simulink model "Copy_of_UAV"  (R2018b)
settings: Solver=FixedStepAuto  StartTime=0  StopTime=300  MaxStep=0.01  RelTol=1e-4  EnableMultiTasking=on
values from neighbouring files (symbols this model uses):
  actuatorCentres = 0.0    [data.sldd]
  datcom1 : value not decoded    [data.sldd]
  deflectionLimits = -10.0    [data.sldd]
  loggingSampleTime = 1.0    [data.sldd]
  sensorSampleTime = 0.02    [data.sldd]
  vehicle = 1.5    [data.sldd]
undefined symbols (not defined in the file or in its folder): aeroCoeff, DiscIntNeverNeededParam, Discrete, HDBK, MIL, Time
libraries: simulink x24, arduinolib x8, ctrlSharedLib x8, aerolibasang x5, aerolibactuator x4, aerolibadyn x3, aerolibconvert2 x2, aerolibatmos2 x2, aerolibnav x2, shared6dof x1, aerolibwind2 x1, simulink_extras x1
(part 2 of 3)

== system Copy_of_UAV/Flight Dynamics/Coeff Model/Aerodynamic Coefficients/Body Rate Damping ==
  V : Inport  Unit=m/s
  Bus Element In : Inport  Port=2  PortName=pqr  Element=p_wind
  Bus Element In1 : Inport  Port=2  PortName=pqr  Element=q_wind
  Bus Element In2 : Inport  Port=2  PortName=pqr  Element=r_wind
  Product : Product  SaturateOnIntegerOverflow=on  InputSameDT=on  OutDataTypeStr=Inherit: Same as first input
  Product1 : Product  SaturateOnIntegerOverflow=on  InputSameDT=on  OutDataTypeStr=Inherit: Same as first input
  Product2 : Product  SaturateOnIntegerOverflow=on  InputSameDT=on  OutDataTypeStr=Inherit: Same as first input
  Product3 : Product  Inputs=*/  SaturateOnIntegerOverflow=on  InputSameDT=on  OutDataTypeStr=Inherit: Same as first input
  Reference Length : Gain  Gain=vehicle.chord  SaturateOnIntegerOverflow=on  OutDataTypeStr=Inherit: Same as input  ParamDataTypeStr=Inherit: Same as input
  Reference Span : Gain  Gain=vehicle.wingspan/2  SaturateOnIntegerOverflow=on  OutDataTypeStr=Inherit: Same as input  ParamDataTypeStr=Inherit: Same as input
  "Reference Span " : Gain  Gain=vehicle.wingspan/2  SaturateOnIntegerOverflow=on  OutDataTypeStr=Inherit: Same as input  ParamDataTypeStr=Inherit: Same as input
  Sum1 : Sum  Inputs=+++  SaturateOnIntegerOverflow=on  InputSameDT=on  OutDataTypeStr=Inherit: Same as first input
  p : Subsystem
  q : Subsystem
  r : Subsystem
  Coeff : Outport  InitialOutput=0
  wires:
  Bus Element In/1 -> Product/2
  Bus Element In1/1 -> Product1/2
  Bus Element In2/1 -> Product2/2
  p/1(delCoeff) -> Product/1
  q/1(delCoeff) -> Product1/1
  Sum1/1 -> Product3/1
  V/1 -> Product3/2
  Product3/1 -> Coeff/1
  Product1/1 -> Reference Length/1
  Product2/1 -> "Reference Span "/1
  Product/1 -> Reference Span/1
  r/1(delCoeff) -> Product2/1
  Reference Length/1 -> Sum1/2
  Reference Span/1 -> Sum1/1
  "Reference Span "/1 -> Sum1/3

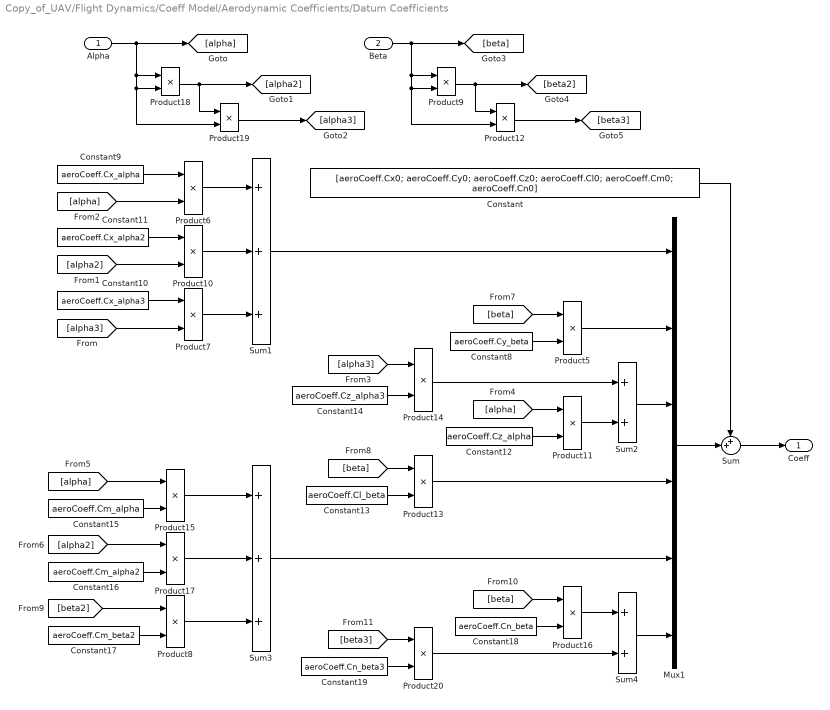
== system Copy_of_UAV/Flight Dynamics/Coeff Model/Aerodynamic Coefficients/Datum Coefficients ==
  Alpha : Inport
  Beta : Inport  Port=2
  Constant : Constant  Value=[aeroCoeff.Cx0; aeroCoeff.Cy0; aeroCoeff.Cz0; aeroCoeff.Cl0; aeroCoeff.Cm0; aeroCoeff.Cn0]
  Constant10 : Constant  Value=aeroCoeff.Cx_alpha3
  Constant11 : Constant  Value=aeroCoeff.Cx_alpha2
  Constant12 : Constant  Value=aeroCoeff.Cz_alpha
  Constant13 : Constant  Value=aeroCoeff.Cl_beta
  Constant14 : Constant  Value=aeroCoeff.Cz_alpha3
  Constant15 : Constant  Value=aeroCoeff.Cm_alpha
  Constant16 : Constant  Value=aeroCoeff.Cm_alpha2
  Constant17 : Constant  Value=aeroCoeff.Cm_beta2
  Constant18 : Constant  Value=aeroCoeff.Cn_beta
  Constant19 : Constant  Value=aeroCoeff.Cn_beta3
  Constant8 : Constant  Value=aeroCoeff.Cy_beta
  Constant9 : Constant  Value=aeroCoeff.Cx_alpha
  Mux1 : Mux  Inputs=6
  Product{5..20} (16 alike) : Product  SaturateOnIntegerOverflow=on  InputSameDT=on  OutDataTypeStr=Inherit: Same as first input
  Sum : Sum  Inputs=++|
  Sum1 : Sum  Inputs=+++  SaturateOnIntegerOverflow=on
  Sum2 : Sum  Inputs=2  SaturateOnIntegerOverflow=on
  Sum3 : Sum  Inputs=+++  SaturateOnIntegerOverflow=on
  Sum4 : Sum  Inputs=2  SaturateOnIntegerOverflow=on
  Coeff : Outport  InitialOutput=0
  wires:
  Sum/1 -> Coeff/1
  Constant/1 -> Sum/1
  Mux1/1 -> Sum/2
  Sum3/1 -> Mux1/5
  Product16/1 -> Sum4/1
  Product20/1 -> Sum4/2
  [beta3] -> Product20/1
  [beta] -> Product16/1
  Constant19/1 -> Product20/2
  Constant18/1 -> Product16/2
  Sum4/1 -> Mux1/6
  [beta2] -> Product8/1
  [beta] -> Product13/1
  [beta] -> Product5/1
  Beta/1 -> Product9/1, Product12/2, Product9/2, [beta]
  Product9/1 -> Product12/1, [beta2]
  Product12/1 -> [beta3]
  Product8/1 -> Sum3/3
  Constant17/1 -> Product8/2
  [alpha] -> Product15/1
  [alpha] -> Product11/1
  [alpha3] -> Product14/1
  [alpha] -> Product6/2
  [alpha2] -> Product10/2
  Constant10/1 -> Product7/1
  [alpha3] -> Product7/2
  Product19/1 -> [alpha3]
  Product18/1 -> [alpha2], Product19/1
  Alpha/1 -> [alpha], Product18/2, Product19/2, Product18/1
  Constant16/1 -> Product17/2
  Product17/1 -> Sum3/2
  [alpha2] -> Product17/1
  Constant15/1 -> Product15/2
  Product15/1 -> Sum3/1
  Constant14/1 -> Product14/2
  Product13/1 -> Mux1/4
  Constant13/1 -> Product13/2
  Sum2/1 -> Mux1/3
  Product14/1 -> Sum2/1
  Product11/1 -> Sum2/2
  Constant12/1 -> Product11/2
  Product10/1 -> Sum1/2
  Product6/1 -> Sum1/1
  Product7/1 -> Sum1/3
  Constant11/1 -> Product10/1
  Constant9/1 -> Product6/1
  Sum1/1 -> Mux1/1
  Product5/1 -> Mux1/2
  Constant8/1 -> Product5/2

== system Copy_of_UAV/Flight Dynamics/DATCOM Model/Aero Coeffs/Aileron ==
  Bus : Inport
  Bus Selector2 : BusSelector  OutputSignals=idxa,fa,idxda,fda,idxm,fm,idxh,fh
  Bus Selector3 : BusSelector  OutputSignals=idxda,fda,idxm,fm,idxh,fh
  Constant1 : Constant  Value=0
  DCL_Roll : Interpolation_n-D  NumberOfTableDimensions=3  Table="permute(datcom1{2}.clroll,[1  2  3])"  RemoveProtectionIndex=on
      settings: InputPortMap=u0,u1,u2,u3,u4,u5
  DCN_Asym : Interpolation_n-D  NumberOfTableDimensions=4  Table=permute(datcom1{2}.cn_asy,[1 2 3 4 ])  RemoveProtectionIndex=on
      settings: InputPortMap=u0,u1,u2,u3,u4,u5,u6,u7
  Mux1 : Mux  Inputs=6
  delCoeff : Outport
  wires:
  Mux1/1 -> delCoeff/1
  Bus Selector3/5 -> DCL_Roll/5  "<idxh>"
  Constant1/1 -> Mux1/1, Mux1/2, Mux1/3, Mux1/5
  Bus Selector3/4 -> DCL_Roll/4  "<fm>"
  Bus Selector3/3 -> DCL_Roll/3  "<idxm>"
  Bus Selector3/6 -> DCL_Roll/6  "<fh>"
  Bus Selector3/1 -> DCL_Roll/1  "<idxda>"
  Bus Selector3/2 -> DCL_Roll/2  "<fda>"
  Bus Selector2/2 -> DCN_Asym/2  "<fa>"
  Bus Selector2/1 -> DCN_Asym/1  "<idxa>"
  Bus/1 -> Bus Selector2/1, Bus Selector3/1
  Bus Selector2/3 -> DCN_Asym/3  "<idxda>"
  Bus Selector2/4 -> DCN_Asym/4  "<fda>"
  Bus Selector2/5 -> DCN_Asym/5  "<idxm>"
  Bus Selector2/6 -> DCN_Asym/6  "<fm>"
  Bus Selector2/7 -> DCN_Asym/7  "<idxh>"
  Bus Selector2/8 -> DCN_Asym/8  "<fh>"
  DCN_Asym/1 -> Mux1/6
  DCL_Roll/1 -> Mux1/4

== system Copy_of_UAV/Flight Dynamics/DATCOM Model/Aero Coeffs/Elevator ==
  Bus : Inport
  Bus Selector2 : BusSelector  OutputSignals=idxa,fa,idxm,fm,idxh,fh,idxde,fde
  Bus Selector3 : BusSelector  OutputSignals=idxde,fde,idxm,fm,idxh,fh
  Bus Selector5 : BusSelector  OutputSignals=idxde,fde,idxm,fm,idxh,fh
  Constant1 : Constant  Value=0
  DCDI : Interpolation_n-D  NumberOfTableDimensions=4  Table=permute(datcom1{3}.dcdi_sym,[1 3 4 2 ])  RemoveProtectionIndex=on
      settings: InputPortMap=u0,u1,u2,u3,u4,u5,u6,u7
  DCL : Interpolation_n-D  NumberOfTableDimensions=3  Table="permute(datcom1{3}.dcl_sym,[1  2  3])"  RemoveProtectionIndex=on
      settings: InputPortMap=u0,u1,u2,u3,u4,u5
  DCm : Interpolation_n-D  NumberOfTableDimensions=3  Table="permute(datcom1{3}.dcm_sym,[1  2  3])"  RemoveProtectionIndex=on
      settings: InputPortMap=u0,u1,u2,u3,u4,u5
  Mux1 : Mux  Inputs=6
  delCoeff : Outport
  wires:
  Mux1/1 -> delCoeff/1
  Bus/1 -> Bus Selector2/1, Bus Selector3/1, Bus Selector5/1
  DCDI/1 -> Mux1/1
  DCL/1 -> Mux1/3
  DCm/1 -> Mux1/5
  Constant1/1 -> Mux1/2, Mux1/4, Mux1/6
  Bus Selector2/1 -> DCDI/1  "<idxa>"
  Bus Selector2/2 -> DCDI/2  "<fa>"
  Bus Selector3/1 -> DCL/1  "<idxde>"
  Bus Selector3/2 -> DCL/2  "<fde>"
  Bus Selector5/1 -> DCm/1  "<idxde>"
  Bus Selector5/2 -> DCm/2  "<fde>"
  Bus Selector2/3 -> DCDI/3  "<idxm>"
  Bus Selector2/4 -> DCDI/4  "<fm>"
  Bus Selector2/5 -> DCDI/5  "<idxh>"
  Bus Selector2/6 -> DCDI/6  "<fh>"
  Bus Selector2/7 -> DCDI/7  "<idxde>"
  Bus Selector2/8 -> DCDI/8  "<fde>"
  Bus Selector3/3 -> DCL/3  "<idxm>"
  Bus Selector3/4 -> DCL/4  "<fm>"
  Bus Selector3/5 -> DCL/5  "<idxh>"
  Bus Selector3/6 -> DCL/6  "<fh>"
  Bus Selector5/3 -> DCm/3  "<idxm>"
  Bus Selector5/4 -> DCm/4  "<fm>"
  Bus Selector5/5 -> DCm/5  "<idxh>"
  Bus Selector5/6 -> DCm/6  "<fh>"

== system Copy_of_UAV/Flight Dynamics/DATCOM Model/Aero Coeffs/Rudder ==
  Bus : Inport
  Constant1 : Constant  Value=0
  Mux1 : Mux  Inputs=6
  Terminator : Terminator
  delCoeff : Outport
  wires:
  Mux1/1 -> delCoeff/1
  Constant1/1 -> Mux1/6, Mux1/5, Mux1/4, Mux1/3, Mux1/2, Mux1/1
  Bus/1 -> Terminator/1

== system Copy_of_UAV/Primary Arduino/Flight Control/Model Flight Control/Guidance/Guidance.ALT_Hold.ALT ==
  Sensors : Inport  OutDataTypeStr=Bus: Sensors
  Demands : Inport  Port=2  OutDataTypeStr=Bus: Demands
  Control Override : Inport  Port=3  OutDataTypeStr=Bus: ControlOverrides
  Action Port : ActionPort
      settings: CopyFcn=Stateflow.SLINSF.SimulinkMan.removeBlockPreDeleteFcn  PreDeleteFcn=Stateflow.SLINSF.SimulinkMan.unsafePredeleteFcn
  Altitude Hold : Subsystem
  Bus Selector : BusSelector  OutputSignals=Altitude,phi_theta_psi
  Bus Selector1 : BusSelector  OutputSignals=Altitude
  Bus Selector2 : BusSelector  OutputSignals=Aileron
  Mux : Mux  Inputs=2
  Rate Limiter : RateLimiter  SampleTimeMode=inherited
  Selector2 : Selector  IndexMode=Zero-based  InputPortWidth=3  IndexOptions=Index vector (dialog)  Indices=[1]  OutputSizes=1
  Commands : Outport
  wires:
  Mux/1 -> Commands/1
  Altitude Hold/1(Elevator) -> Mux/2
  Selector2/1 -> Altitude Hold/3(theta)
  Sensors/1 -> Bus Selector/1
  Demands/1 -> Bus Selector1/1
  Bus Selector/1 -> Altitude Hold/1(ALT)  "<Altitude>"
  Bus Selector/2 -> Selector2/1  "<phi_theta_psi>"
  Bus Selector1/1 -> Rate Limiter/1  "<Altitude>"
  Rate Limiter/1 -> Altitude Hold/2(Demanded ALT)
  Bus Selector2/1 -> Mux/1  "<Aileron>"
  Control Override/1 -> Bus Selector2/1

== system Copy_of_UAV/Primary Arduino/Flight Control/Model Flight Control/Guidance/Guidance.HDG_ALT_Hold.HDG_ALT ==
  Sensors : Inport  OutDataTypeStr=Bus: Sensors
  Demands : Inport  Port=2  OutDataTypeStr=Bus: Demands
  Action Port : ActionPort
      settings: CopyFcn=Stateflow.SLINSF.SimulinkMan.removeBlockPreDeleteFcn  PreDeleteFcn=Stateflow.SLINSF.SimulinkMan.unsafePredeleteFcn
  Altitude Hold : Subsystem
      settings: UndoDeleteFcn=Stateflow.SLINSF.SimulinkMan.restorePreDeleteFcn  PreDeleteFcn=Stateflow.SLINSF.SimulinkMan.removePreDeleteFcn
  Bus Selector : BusSelector  OutputSignals=Heading,phi_theta_psi,Altitude
  Bus Selector1 : BusSelector  OutputSignals=Heading,Altitude
  Heading Hold : Subsystem
  Mux : Mux  Inputs=2
  Rate Limiter : RateLimiter  SampleTimeMode=inherited
  Rate Limiter1 : RateLimiter  SampleTimeMode=inherited
  Selector : Selector  IndexMode=Zero-based  InputPortWidth=3  IndexOptions=Index vector (dialog)  Indices=[0]  OutputSizes=1
  Selector2 : Selector  IndexMode=Zero-based  InputPortWidth=3  IndexOptions=Index vector (dialog)  Indices=[1]  OutputSizes=1
  Commands : Outport
  wires:
  Heading Hold/1(Aileron) -> Mux/1  "Aileron"
  Mux/1 -> Commands/1
  Altitude Hold/1(Elevator) -> Mux/2  "Elevator"
  Selector2/1 -> Altitude Hold/3(theta)
  Sensors/1 -> Bus Selector/1
  Selector/1 -> Heading Hold/3(Current Roll Angle)
  Demands/1 -> Bus Selector1/1
  Bus Selector/3 -> Altitude Hold/1(ALT)  "<Altitude>"
  Bus Selector1/1 -> Rate Limiter/1  "<Heading>"
  Bus Selector/1 -> Heading Hold/1(Current Heading)  "<Heading>"
  Bus Selector/2 -> Selector2/1, Selector/1  "<phi_theta_psi>"
  Bus Selector1/2 -> Rate Limiter1/1  "<Altitude>"
  Rate Limiter/1 -> Heading Hold/2(Demanded Heading)
  Rate Limiter1/1 -> Altitude Hold/2(ALT Demand)

== system Copy_of_UAV/Primary Arduino/Flight Control/Model Flight Control/Guidance/Guidance.HDG_Hold.HDG ==
  Sensors : Inport  OutDataTypeStr=Bus: Sensors
  Demands : Inport  Port=2  OutDataTypeStr=Bus: Demands
  Control Override : Inport  Port=3  OutDataTypeStr=Bus: ControlOverrides
  Action Port : ActionPort
      settings: CopyFcn=Stateflow.SLINSF.SimulinkMan.removeBlockPreDeleteFcn  PreDeleteFcn=Stateflow.SLINSF.SimulinkMan.unsafePredeleteFcn
  Bus Selector : BusSelector  OutputSignals=Heading,phi_theta_psi
  Bus Selector1 : BusSelector  OutputSignals=Heading
  Bus Selector2 : BusSelector  OutputSignals=Elevator
  Heading Hold : Subsystem
  Mux : Mux  Inputs=2
  Rate Limiter : RateLimiter  SampleTimeMode=inherited
  Selector : Selector  IndexMode=Zero-based  InputPortWidth=3  IndexOptions=Index vector (dialog)  Indices=[0]  OutputSizes=1
  Command : Outport
  wires:
  Heading Hold/1(Aileron Command) -> Mux/1  "Aileron"
  Sensors/1 -> Bus Selector/1
  Selector/1 -> Heading Hold/3(Current Roll Angle)
  Demands/1 -> Bus Selector1/1
  Bus Selector1/1 -> Rate Limiter/1  "<Heading>"
  Bus Selector/1 -> Heading Hold/1(Current Heading)  "<Heading>"
  Bus Selector/2 -> Selector/1  "<phi_theta_psi>"
  Rate Limiter/1 -> Heading Hold/2(Demanded Heading)
  Mux/1 -> Command/1
  Control Override/1 -> Bus Selector2/1
  Bus Selector2/1 -> Mux/2  "<Elevator>"

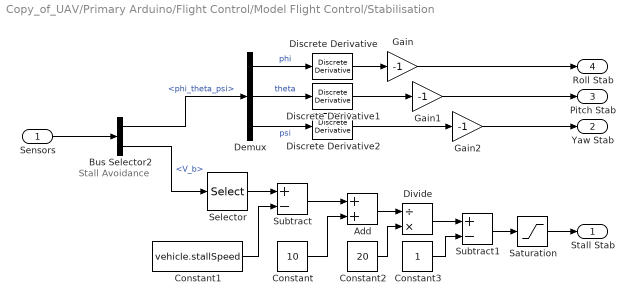
== system Copy_of_UAV/Primary Arduino/Flight Control/Model Flight Control/Stabilisation ==
  note: Stall Avoidance
  Sensors : Inport
  Add : Sum
  Bus Selector2 : BusSelector  OutputSignals=phi_theta_psi,V_b
  Constant : Constant  Value=10  OutDataTypeStr=single
  Constant1 : Constant  Value=vehicle.stallSpeed  OutDataTypeStr=single
  Constant2 : Constant  Value=20  OutDataTypeStr=single
  Constant3 : Constant  OutDataTypeStr=single
  Demux : Demux  Outputs=3
  Discrete Derivative : simulink/Discrete/Discrete Derivative  gainval=1.0  ICPrevScaledInput=0.0  OutMin=[]  OutMax=[]  OutDataType=fixdt(1, 16)  OutScaling=2^-10  DoSatur=off
  Discrete Derivative1 : simulink/Discrete/Discrete Derivative  gainval=1.0  ICPrevScaledInput=0.0  OutMin=[]  OutMax=[]  OutDataType=fixdt(1, 16)  OutScaling=2^-10  DoSatur=off
  Discrete Derivative2 : simulink/Discrete/Discrete Derivative  gainval=1.0  ICPrevScaledInput=0.0  OutMin=[]  OutMax=[]  OutDataType=fixdt(1, 16)  OutScaling=2^-10  DoSatur=off
  Divide : Product  Inputs=/*
  Gain : Gain  Gain=-1
  Gain1 : Gain  Gain=-1
  Gain2 : Gain  Gain=-1
  Saturation : Saturate  UpperLimit=1  LowerLimit=0
  Selector : Selector  IndexMode=Zero-based  InputPortWidth=3  IndexOptions=Index vector (dialog)  Indices=[0]  OutputSizes=1
  Subtract : Sum  Inputs=+-
  Subtract1 : Sum  Inputs=+-
  Stall Stab : Outport
  Yaw Stab : Outport  Port=2
  Pitch Stab : Outport  Port=3
  Roll Stab : Outport  Port=4
  wires:
  Gain2/1 -> Yaw Stab/1
  Bus Selector2/2 -> Selector/1  "<V_b>"
  Discrete Derivative2/1 -> Gain2/1
  Selector/1 -> Subtract/1
  Sensors/1 -> Bus Selector2/1
  Demux/2 -> Discrete Derivative1/1  "theta"
  Demux/1 -> Discrete Derivative/1  "phi"
  Demux/3 -> Discrete Derivative2/1  "psi"
  Discrete Derivative1/1 -> Gain1/1
  Discrete Derivative/1 -> Gain/1
  Bus Selector2/1 -> Demux/1  "<phi_theta_psi>"
  Gain/1 -> Roll Stab/1
  Gain1/1 -> Pitch Stab/1
  Constant1/1 -> Subtract/2
  Saturation/1 -> Stall Stab/1
  Subtract/1 -> Add/1
  Constant/1 -> Add/2
  Add/1 -> Divide/1
  Constant2/1 -> Divide/2
  Divide/1 -> Subtract1/1
  Constant3/1 -> Subtract1/2
  Subtract1/1 -> Saturation/1

== system Copy_of_UAV/Primary Arduino/Flight Control/Real Flight Control/Guidance/Guidance.ALT_Hold.ALT ==
  Sensors : Inport  OutDataTypeStr=Bus: Sensors
  Demands : Inport  Port=2  OutDataTypeStr=Bus: Demands
  Action Port : ActionPort
      settings: CopyFcn=Stateflow.SLINSF.SimulinkMan.removeBlockPreDeleteFcn  PreDeleteFcn=Stateflow.SLINSF.SimulinkMan.unsafePredeleteFcn
  Altitude Hold : Subsystem
  Bus Selector : BusSelector  OutputSignals=Altitude,phi_theta_psi
  Bus Selector1 : BusSelector  OutputSignals=Altitude
  Constant : Constant  Value=0
  Mux : Mux  Inputs=2
  Rate Limiter : RateLimiter  SampleTimeMode=inherited
  Selector2 : Selector  IndexMode=Zero-based  InputPortWidth=3  IndexOptions=Index vector (dialog)  Indices=[1]  OutputSizes=1
  Commands : Outport
  wires:
  Mux/1 -> Commands/1
  Altitude Hold/1(Elevator) -> Mux/2
  Selector2/1 -> Altitude Hold/3(theta)
  Sensors/1 -> Bus Selector/1
  Demands/1 -> Bus Selector1/1
  Bus Selector/1 -> Altitude Hold/1(ALT)  "<Altitude>"
  Bus Selector/2 -> Selector2/1  "<phi_theta_psi>"
  Bus Selector1/1 -> Rate Limiter/1  "<Altitude>"
  Rate Limiter/1 -> Altitude Hold/2(Demanded ALT)
  Constant/1 -> Mux/1

== system Copy_of_UAV/Primary Arduino/Flight Control/Real Flight Control/Guidance/Guidance.HDG_ALT_Hold.HDG_ALT ==
  Sensors : Inport  OutDataTypeStr=Bus: Sensors
  Demands : Inport  Port=2  OutDataTypeStr=Bus: Demands
  Action Port : ActionPort
      settings: CopyFcn=Stateflow.SLINSF.SimulinkMan.removeBlockPreDeleteFcn  PreDeleteFcn=Stateflow.SLINSF.SimulinkMan.unsafePredeleteFcn
  Altitude Hold : Subsystem
      settings: UndoDeleteFcn=Stateflow.SLINSF.SimulinkMan.restorePreDeleteFcn  PreDeleteFcn=Stateflow.SLINSF.SimulinkMan.removePreDeleteFcn
  Bus Selector : BusSelector  OutputSignals=Heading,phi_theta_psi,Altitude
  Bus Selector1 : BusSelector  OutputSignals=Heading,Altitude
  Heading Hold : Subsystem
  Mux : Mux  Inputs=2
  Rate Limiter : RateLimiter  SampleTimeMode=inherited
  Rate Limiter1 : RateLimiter  SampleTimeMode=inherited
  Selector : Selector  IndexMode=Zero-based  InputPortWidth=3  IndexOptions=Index vector (dialog)  Indices=[0]  OutputSizes=1
  Selector2 : Selector  IndexMode=Zero-based  InputPortWidth=3  IndexOptions=Index vector (dialog)  Indices=[1]  OutputSizes=1
  Commands : Outport
  wires:
  Heading Hold/1(Aileron) -> Mux/1  "Aileron"
  Mux/1 -> Commands/1
  Altitude Hold/1(Elevator) -> Mux/2  "Elevator"
  Selector2/1 -> Altitude Hold/3(theta)
  Sensors/1 -> Bus Selector/1
  Selector/1 -> Heading Hold/3(Current Roll Angle)
  Demands/1 -> Bus Selector1/1
  Bus Selector/3 -> Altitude Hold/1(ALT)  "<Altitude>"
  Bus Selector1/1 -> Rate Limiter/1  "<Heading>"
  Bus Selector/1 -> Heading Hold/1(Current Heading)  "<Heading>"
  Bus Selector/2 -> Selector2/1, Selector/1  "<phi_theta_psi>"
  Bus Selector1/2 -> Rate Limiter1/1  "<Altitude>"
  Rate Limiter/1 -> Heading Hold/2(Demanded Heading)
  Rate Limiter1/1 -> Altitude Hold/2(ALT Demand)

== system Copy_of_UAV/Primary Arduino/Flight Control/Real Flight Control/Guidance/Guidance.HDG_Hold.HDG ==
  Sensors : Inport  OutDataTypeStr=Bus: Sensors
  Demands : Inport  Port=2  OutDataTypeStr=Bus: Demands
  Action Port : ActionPort
      settings: CopyFcn=Stateflow.SLINSF.SimulinkMan.removeBlockPreDeleteFcn  PreDeleteFcn=Stateflow.SLINSF.SimulinkMan.unsafePredeleteFcn
  Bus Selector : BusSelector  OutputSignals=Heading,phi_theta_psi
  Bus Selector1 : BusSelector  OutputSignals=Heading
  Constant : Constant  Value=0
  Heading Hold : Subsystem
  Mux : Mux  Inputs=2
  Rate Limiter : RateLimiter  SampleTimeMode=inherited
  Selector : Selector  IndexMode=Zero-based  InputPortWidth=3  IndexOptions=Index vector (dialog)  Indices=[0]  OutputSizes=1
  Command : Outport
  wires:
  Heading Hold/1(Aileron Command) -> Mux/1  "Aileron"
  Sensors/1 -> Bus Selector/1
  Selector/1 -> Heading Hold/3(Current Roll Angle)
  Demands/1 -> Bus Selector1/1
  Bus Selector1/1 -> Rate Limiter/1  "<Heading>"
  Bus Selector/1 -> Heading Hold/1(Current Heading)  "<Heading>"
  Bus Selector/2 -> Selector/1  "<phi_theta_psi>"
  Rate Limiter/1 -> Heading Hold/2(Demanded Heading)
  Mux/1 -> Command/1
  Constant/1 -> Mux/2

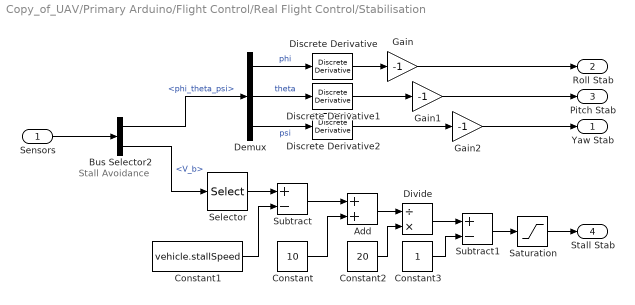
== system Copy_of_UAV/Primary Arduino/Flight Control/Real Flight Control/Stabilisation ==
  note: Stall Avoidance
  Sensors : Inport
  Add : Sum
  Bus Selector2 : BusSelector  OutputSignals=phi_theta_psi,V_b
  Constant : Constant  Value=10  OutDataTypeStr=single
  Constant1 : Constant  Value=vehicle.stallSpeed  OutDataTypeStr=single
  Constant2 : Constant  Value=20  OutDataTypeStr=single
  Constant3 : Constant  OutDataTypeStr=single
  Demux : Demux  Outputs=3
  Discrete Derivative : simulink/Discrete/Discrete Derivative  gainval=1.0  ICPrevScaledInput=0.0  OutMin=[]  OutMax=[]  OutDataType=fixdt(1, 16)  OutScaling=2^-10  DoSatur=off
  Discrete Derivative1 : simulink/Discrete/Discrete Derivative  gainval=1.0  ICPrevScaledInput=0.0  OutMin=[]  OutMax=[]  OutDataType=fixdt(1, 16)  OutScaling=2^-10  DoSatur=off
  Discrete Derivative2 : simulink/Discrete/Discrete Derivative  gainval=1.0  ICPrevScaledInput=0.0  OutMin=[]  OutMax=[]  OutDataType=fixdt(1, 16)  OutScaling=2^-10  DoSatur=off
  Divide : Product  Inputs=/*
  Gain : Gain  Gain=-1
  Gain1 : Gain  Gain=-1
  Gain2 : Gain  Gain=-1
  Saturation : Saturate  UpperLimit=1  LowerLimit=0
  Selector : Selector  IndexMode=Zero-based  InputPortWidth=3  IndexOptions=Index vector (dialog)  Indices=[0]  OutputSizes=1
  Subtract : Sum  Inputs=+-
  Subtract1 : Sum  Inputs=+-
  Yaw Stab : Outport
  Roll Stab : Outport  Port=2
  Pitch Stab : Outport  Port=3
  Stall Stab : Outport  Port=4
  wires:
  Gain2/1 -> Yaw Stab/1
  Bus Selector2/2 -> Selector/1  "<V_b>"
  Discrete Derivative2/1 -> Gain2/1
  Selector/1 -> Subtract/1
  Sensors/1 -> Bus Selector2/1
  Demux/2 -> Discrete Derivative1/1  "theta"
  Demux/1 -> Discrete Derivative/1  "phi"
  Demux/3 -> Discrete Derivative2/1  "psi"
  Discrete Derivative1/1 -> Gain1/1
  Discrete Derivative/1 -> Gain/1
  Bus Selector2/1 -> Demux/1  "<phi_theta_psi>"
  Gain/1 -> Roll Stab/1
  Gain1/1 -> Pitch Stab/1
  Constant1/1 -> Subtract/2
  Saturation/1 -> Stall Stab/1
  Subtract/1 -> Add/1
  Constant/1 -> Add/2
  Add/1 -> Divide/1
  Constant2/1 -> Divide/2
  Divide/1 -> Subtract1/1
  Constant3/1 -> Subtract1/2
  Subtract1/1 -> Saturation/1

== system Copy_of_UAV/Primary Arduino/Sensors/Sensor Hardware/Model Sensors ==
  States : Inport
  Add : Sum
  "BMP280 PAT Sensor " : Subsystem
  Bus Selector : BusSelector  OutputSignals=X_e,phi_theta_psi,pqr,A_be,omega_dot
  Constant2 : Constant  Value=9.81  OutDataTypeStr=single
  Constant3 : Constant  Value=vehicle.CG  OutDataTypeStr=single
  Constant4 : Constant  OutDataTypeStr=single
  Divide1 : Product  Inputs=*/
  L3GD20 3 Axis Gyro Sensor : Subsystem
  LSM303 Accel + Compass Sensor : Subsystem
  Pressure_Pa : Outport
  Temp_C : Outport  Port=2
  RotVel : Outport  Port=3
  LinAccel : Outport  Port=4
  Heading : Outport  Port=5
  Altitude : Outport  Port=6
  wires:
  Constant3/1 -> LSM303 Accel + Compass Sensor/4(CoG)
  Constant4/1 -> Add/2
  Bus Selector/1 -> "BMP280 PAT Sensor "/1(X_e)  "<X_e>"
  Constant2/1 -> Divide1/2
  Bus Selector/4 -> LSM303 Accel + Compass Sensor/1(A_b), Divide1/1  "<A_be>"
  Bus Selector/3 -> LSM303 Accel + Compass Sensor/2(omega), L3GD20 3 Axis Gyro Sensor/1(omega)  "<pqr>"
  L3GD20 3 Axis Gyro Sensor/1(RotVel) -> RotVel/1  "RotVel"
  Add/1 -> L3GD20 3 Axis Gyro Sensor/2(G's)
  Divide1/1 -> Add/1
  "BMP280 PAT Sensor "/3(Altitude_m) -> Altitude/1  "Altitude"
  Bus Selector/2 -> LSM303 Accel + Compass Sensor/5(phi_theta_psi)  "<phi_theta_psi>"
  Bus Selector/5 -> LSM303 Accel + Compass Sensor/3(omega_dot)  "<omega_dot>"
  LSM303 Accel + Compass Sensor/1(LinAccel) -> LinAccel/1  "LinAccel"
  "BMP280 PAT Sensor "/1(Pressure_Pa) -> Pressure_Pa/1  "Pressure_Pa"
  States/1 -> Bus Selector/1
  "BMP280 PAT Sensor "/2(Temp_C) -> Temp_C/1  "Temp_C"
  LSM303 Accel + Compass Sensor/2(hdg_deg) -> Heading/1  "Heading"

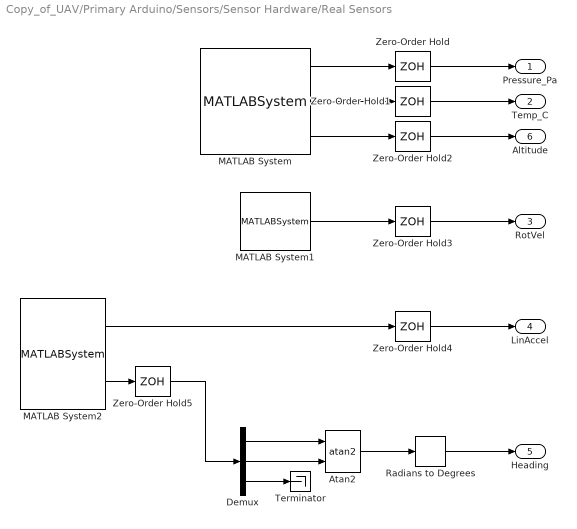
== system Copy_of_UAV/Primary Arduino/Sensors/Sensor Hardware/Real Sensors ==
  Atan2 : Trigonometry  Operator=atan2
  Demux : Demux  Outputs=3
  MATLAB System : MATLABSystem  System=BMP085  Reference_Pressure=101325  SimulateUsing=Code generation
      mask Type: BMP085
      mask Display:
      | disp('BMP085');
      | port_label('output',1,'press');
      | port_label('output',2,'temp');
      | port_label('output',3,'alt');
  MATLAB System1 : MATLABSystem  System=L3GD20  SimulateUsing=Code generation
      mask Type: L3GD20
      mask Display:
      | disp('L3GD20');
      | port_label('output',1,'rot');
  MATLAB System2 : MATLABSystem  System=LSM303  SimulateUsing=Code generation
      mask Type: LSM303
      mask Display:
      | disp('LSM303');
      | port_label('output',1,'accel');
      | port_label('output',2,'mag');
  Radians to Degrees : simulink_extras/Transformations/Radians to Degrees
  Terminator : Terminator
  Zero-Order Hold{,1..5} (6 alike) : ZeroOrderHold  SampleTime=sensorSampleTime
  Pressure_Pa : Outport
  Temp_C : Outport  Port=2
  RotVel : Outport  Port=3
  LinAccel : Outport  Port=4
  Heading : Outport  Port=5
  Altitude : Outport  Port=6
  wires:
  Zero-Order Hold/1 -> Pressure_Pa/1
  Zero-Order Hold1/1 -> Temp_C/1
  Zero-Order Hold2/1 -> Altitude/1
  Zero-Order Hold3/1 -> RotVel/1
  Zero-Order Hold4/1 -> LinAccel/1
  MATLAB System/1 -> Zero-Order Hold/1
  MATLAB System/2 -> Zero-Order Hold1/1
  MATLAB System/3 -> Zero-Order Hold2/1
  MATLAB System1/1 -> Zero-Order Hold3/1
  MATLAB System2/1 -> Zero-Order Hold4/1
  MATLAB System2/2 -> Zero-Order Hold5/1
  Zero-Order Hold5/1 -> Demux/1
  Demux/1 -> Atan2/1
  Demux/2 -> Atan2/2
  Atan2/1 -> Radians to Degrees/1
  Radians to Degrees/1 -> Heading/1
  Demux/3 -> Terminator/1

== system Copy_of_UAV/Flight Dynamics/Coeff Model/Aerodynamic Coefficients/Body Rate Damping/p ==
  Constant1 : Constant  Value=0
  Constant2 : Constant  Value=0
  Constant3 : Constant  Value=0
  Constant4 : Constant  Value=aeroCoeff.Cl_p
  Constant5 : Constant  Value=aeroCoeff.Cn_p
  Constant8 : Constant  Value=aeroCoeff.Cy_p
  Mux1 : Mux  Inputs=6
  delCoeff : Outport
  wires:
  Constant4/1 -> Mux1/4
  Constant5/1 -> Mux1/6
  Constant8/1 -> Mux1/2
  Constant2/1 -> Mux1/3
  Constant3/1 -> Mux1/5
  Constant1/1 -> Mux1/1
  Mux1/1 -> delCoeff/1

== system Copy_of_UAV/Flight Dynamics/Coeff Model/Aerodynamic Coefficients/Body Rate Damping/q ==
  Constant1 : Constant  Value=0
  Constant2 : Constant  Value=0
  Constant3 : Constant  Value=aeroCoeff.Cn_q
  Constant4 : Constant  Value=aeroCoeff.Cz_q
  Constant5 : Constant  Value=aeroCoeff.Cm_q
  Constant8 : Constant  Value=aeroCoeff.Cx_q
  Mux1 : Mux  Inputs=6
  delCoeff : Outport
  wires:
  Constant3/1 -> Mux1/6
  Constant5/1 -> Mux1/5
  Constant4/1 -> Mux1/3
  Constant8/1 -> Mux1/1
  Constant1/1 -> Mux1/2
  Constant2/1 -> Mux1/4
  Mux1/1 -> delCoeff/1

== system Copy_of_UAV/Flight Dynamics/Coeff Model/Aerodynamic Coefficients/Body Rate Damping/r ==
  Constant1 : Constant  Value=0
  Constant2 : Constant  Value=0
  Constant3 : Constant  Value=aeroCoeff.Cm_r
  Constant4 : Constant  Value=aeroCoeff.Cl_r
  Constant5 : Constant  Value=aeroCoeff.Cn_r
  Constant6 : Constant  Value=aeroCoeff.Cy_r
  Mux1 : Mux  Inputs=6
  delCoeff : Outport
  wires:
  Constant6/1 -> Mux1/2
  Constant2/1 -> Mux1/3
  Constant3/1 -> Mux1/5
  Constant5/1 -> Mux1/6
  Constant1/1 -> Mux1/1
  Mux1/1 -> delCoeff/1
  Constant4/1 -> Mux1/4

== system Copy_of_UAV/Primary Arduino/Flight Control/Model Flight Control/Guidance/Guidance.ALT_Hold.ALT/Altitude Hold ==
  ALT : Inport
  Demanded ALT : Inport  Port=2
  theta : Inport  Port=3
  Elevator Controller : simulink/Continuous/PID Controller  Controller=PID  Form=Parallel  TimeDomain=Discrete-time  SampleTime=-1  IntegratorMethod=Forward Euler  FilterMethod=Forward Euler  ControllerParametersSource=internal  P=1  I=1  D=0  UseFilter=on  N=100  TunerSelectOption=Transfer Function Based (PID Tuner App)  InitialConditionSource=internal  InitialConditionForIntegrator=0  InitialConditionForFilter=0  DifferentiatorICPrevScaledInput=0  ExternalReset=none  TrackingMode=off  Kt=1  LimitOutput=off  UpperSaturationLimit=inf  LowerSaturationLimit=-inf  LinearizeAsGain=off  AntiWindupMode=none  Kb=1  POutMin=[]  POutMax=[]  IOutMin=[]  IOutMax=[]  DOutMin=[]  DOutMax=[]  NOutMin=[]  NOutMax=[]  SumOutMin=[]  SumOutMax=[]  SaturationOutMin=[]  SaturationOutMax=[]  PParamMin=[]  PParamMax=[]  IParamMin=[]  IParamMax=[]  DParamMin=[]  DParamMax=[]  NParamMin=[]  NParamMax=[]  KbParamMin=[]  KbParamMax=[]  KtParamMin=[]  KtParamMax=[]  KbOutMin=[]  KbOutMax=[]  KtOutMin=[]  KtOutMax=[]  IntegratorOutMin=[]  IntegratorOutMax=[]  FilterOutMin=[]  FilterOutMax=[]  SumI1OutMin=[]  SumI1OutMax=[]  SumI2OutMin=[]  SumI2OutMax=[]  SumI3OutMin=[]  SumI3OutMax=[]  SumI4OutMin=[]  SumI4OutMax=[]  SumDOutMin=[]  SumDOutMax=[]  DifferentiatorOutMin=[]  DifferentiatorOutMax=[]  FilterDiffOutCoefMin=[]  FilterDiffOutCoefMax=[]  ReciprocalOutMin=[]  ReciprocalOutMax=[]  SumDenOutMin=[]  SumDenOutMax=[]  SumNumOutMin=[]  SumNumOutMax=[]  DivideOutMin=[]  DivideOutMax=[]  IntegratorContinuousStateAttributes=''  IntegratorStateMustResolveToSignalObject=off  IntegratorRTWStateStorageClass=Auto  FilterContinuousStateAttributes=''  FilterStateMustResolveToSignalObject=off  FilterRTWStateStorageClass=Auto  ParallelPVariant=InternalParameters  IdealPVariant=Disabled  IVariant=InternalParameters  DVariant=InternalParameters  IntegratorVariant=Discrete  SatVariant=Disabled  AWVariant=Passthrough  PCopyVariant=Disabled  TRVariant=Disabled  FdbkBlocksVariant=Forward  IdealPFdbkVariant=Disabled  SatFdbkVariant=Disabled  DerivativeFilterVariant=ForwardEulerFilter  NVariant=InternalParameters  NCopyVariant=Disabled  FilterICVariant=InternalICsFilter  IntegratorICVariant=InternalICs  ExternalResetVariant=Disabled  TRSumVariant=Passthrough  SumFdbkVariant=Disabled  SumVariant=Sum_PID
  Pitch Controller : simulink/Continuous/PID Controller  Controller=PID  Form=Parallel  TimeDomain=Discrete-time  SampleTime=-1  IntegratorMethod=Forward Euler  FilterMethod=Forward Euler  ControllerParametersSource=internal  P=1  I=1  D=0  UseFilter=on  N=100  TunerSelectOption=Transfer Function Based (PID Tuner App)  InitialConditionSource=internal  InitialConditionForIntegrator=0  InitialConditionForFilter=0  DifferentiatorICPrevScaledInput=0  ExternalReset=none  TrackingMode=off  Kt=1  LimitOutput=off  UpperSaturationLimit=inf  LowerSaturationLimit=-inf  LinearizeAsGain=off  AntiWindupMode=none  Kb=1  POutMin=[]  POutMax=[]  IOutMin=[]  IOutMax=[]  DOutMin=[]  DOutMax=[]  NOutMin=[]  NOutMax=[]  SumOutMin=[]  SumOutMax=[]  SaturationOutMin=[]  SaturationOutMax=[]  PParamMin=[]  PParamMax=[]  IParamMin=[]  IParamMax=[]  DParamMin=[]  DParamMax=[]  NParamMin=[]  NParamMax=[]  KbParamMin=[]  KbParamMax=[]  KtParamMin=[]  KtParamMax=[]  KbOutMin=[]  KbOutMax=[]  KtOutMin=[]  KtOutMax=[]  IntegratorOutMin=[]  IntegratorOutMax=[]  FilterOutMin=[]  FilterOutMax=[]  SumI1OutMin=[]  SumI1OutMax=[]  SumI2OutMin=[]  SumI2OutMax=[]  SumI3OutMin=[]  SumI3OutMax=[]  SumI4OutMin=[]  SumI4OutMax=[]  SumDOutMin=[]  SumDOutMax=[]  DifferentiatorOutMin=[]  DifferentiatorOutMax=[]  FilterDiffOutCoefMin=[]  FilterDiffOutCoefMax=[]  ReciprocalOutMin=[]  ReciprocalOutMax=[]  SumDenOutMin=[]  SumDenOutMax=[]  SumNumOutMin=[]  SumNumOutMax=[]  DivideOutMin=[]  DivideOutMax=[]  IntegratorContinuousStateAttributes=''  IntegratorStateMustResolveToSignalObject=off  IntegratorRTWStateStorageClass=Auto  FilterContinuousStateAttributes=''  FilterStateMustResolveToSignalObject=off  FilterRTWStateStorageClass=Auto  ParallelPVariant=InternalParameters  IdealPVariant=Disabled  IVariant=InternalParameters  DVariant=InternalParameters  IntegratorVariant=Discrete  SatVariant=Disabled  AWVariant=Passthrough  PCopyVariant=Disabled  TRVariant=Disabled  FdbkBlocksVariant=Forward  IdealPFdbkVariant=Disabled  SatFdbkVariant=Disabled  DerivativeFilterVariant=ForwardEulerFilter  NVariant=InternalParameters  NCopyVariant=Disabled  FilterICVariant=InternalICsFilter  IntegratorICVariant=InternalICs  ExternalResetVariant=Disabled  TRSumVariant=Passthrough  SumFdbkVariant=Disabled  SumVariant=Sum_PID
  Sum : Sum  Inputs=+-
  Sum1 : Sum  Inputs=+-
  Elevator : Outport
  wires:
  Pitch Controller/1 -> Sum1/1
  theta/1 -> Sum1/2
  Demanded ALT/1 -> Sum/2
  Sum/1 -> Pitch Controller/1
  Elevator Controller/1 -> Elevator/1  "Elevator"
  ALT/1 -> Sum/1
  Sum1/1 -> Elevator Controller/1

== system Copy_of_UAV/Primary Arduino/Flight Control/Model Flight Control/Guidance/Guidance.HDG_ALT_Hold.HDG_ALT/Altitude Hold ==
  ALT : Inport
  ALT Demand : Inport  Port=2
  theta : Inport  Port=3
  Altitude Hold : Subsystem
  Elevator : Outport
  wires:
  theta/1 -> Altitude Hold/3(theta)
  ALT Demand/1 -> Altitude Hold/2(In2)
  ALT/1 -> Altitude Hold/1(In1)
  Altitude Hold/1(Elevator) -> Elevator/1

== system Copy_of_UAV/Primary Arduino/Flight Control/Model Flight Control/Guidance/Guidance.HDG_ALT_Hold.HDG_ALT/Heading Hold ==
  Current Heading : Inport
  Demanded Heading : Inport  Port=2
  Current Roll Angle : Inport  Port=3
  Aileron Controller : simulink/Continuous/PID Controller  Controller=PID  Form=Parallel  TimeDomain=Discrete-time  SampleTime=-1  IntegratorMethod=Forward Euler  FilterMethod=Forward Euler  ControllerParametersSource=internal  P=1  I=1  D=0  UseFilter=on  N=100  TunerSelectOption=Transfer Function Based (PID Tuner App)  InitialConditionSource=internal  InitialConditionForIntegrator=0  InitialConditionForFilter=0  DifferentiatorICPrevScaledInput=0  ExternalReset=none  TrackingMode=off  Kt=1  LimitOutput=off  UpperSaturationLimit=inf  LowerSaturationLimit=-inf  LinearizeAsGain=off  AntiWindupMode=none  Kb=1  POutMin=[]  POutMax=[]  IOutMin=[]  IOutMax=[]  DOutMin=[]  DOutMax=[]  NOutMin=[]  NOutMax=[]  SumOutMin=[]  SumOutMax=[]  SaturationOutMin=[]  SaturationOutMax=[]  PParamMin=[]  PParamMax=[]  IParamMin=[]  IParamMax=[]  DParamMin=[]  DParamMax=[]  NParamMin=[]  NParamMax=[]  KbParamMin=[]  KbParamMax=[]  KtParamMin=[]  KtParamMax=[]  KbOutMin=[]  KbOutMax=[]  KtOutMin=[]  KtOutMax=[]  IntegratorOutMin=[]  IntegratorOutMax=[]  FilterOutMin=[]  FilterOutMax=[]  SumI1OutMin=[]  SumI1OutMax=[]  SumI2OutMin=[]  SumI2OutMax=[]  SumI3OutMin=[]  SumI3OutMax=[]  SumI4OutMin=[]  SumI4OutMax=[]  SumDOutMin=[]  SumDOutMax=[]  DifferentiatorOutMin=[]  DifferentiatorOutMax=[]  FilterDiffOutCoefMin=[]  FilterDiffOutCoefMax=[]  ReciprocalOutMin=[]  ReciprocalOutMax=[]  SumDenOutMin=[]  SumDenOutMax=[]  SumNumOutMin=[]  SumNumOutMax=[]  DivideOutMin=[]  DivideOutMax=[]  IntegratorContinuousStateAttributes=''  IntegratorStateMustResolveToSignalObject=off  IntegratorRTWStateStorageClass=Auto  FilterContinuousStateAttributes=''  FilterStateMustResolveToSignalObject=off  FilterRTWStateStorageClass=Auto  ParallelPVariant=InternalParameters  IdealPVariant=Disabled  IVariant=InternalParameters  DVariant=InternalParameters  IntegratorVariant=Discrete  SatVariant=Disabled  AWVariant=Passthrough  PCopyVariant=Disabled  TRVariant=Disabled  FdbkBlocksVariant=Forward  IdealPFdbkVariant=Disabled  SatFdbkVariant=Disabled  DerivativeFilterVariant=ForwardEulerFilter  NVariant=InternalParameters  NCopyVariant=Disabled  FilterICVariant=InternalICsFilter  IntegratorICVariant=InternalICs  ExternalResetVariant=Disabled  TRSumVariant=Passthrough  SumFdbkVariant=Disabled  SumVariant=Sum_PID
  Roll Controller : simulink/Continuous/PID Controller  Controller=PID  Form=Parallel  TimeDomain=Discrete-time  SampleTime=-1  IntegratorMethod=Forward Euler  FilterMethod=Forward Euler  ControllerParametersSource=internal  P=1  I=1  D=0  UseFilter=on  N=100  TunerSelectOption=Transfer Function Based (PID Tuner App)  InitialConditionSource=internal  InitialConditionForIntegrator=0  InitialConditionForFilter=0  DifferentiatorICPrevScaledInput=0  ExternalReset=none  TrackingMode=off  Kt=1  LimitOutput=off  UpperSaturationLimit=inf  LowerSaturationLimit=-inf  LinearizeAsGain=off  AntiWindupMode=none  Kb=1  POutMin=[]  POutMax=[]  IOutMin=[]  IOutMax=[]  DOutMin=[]  DOutMax=[]  NOutMin=[]  NOutMax=[]  SumOutMin=[]  SumOutMax=[]  SaturationOutMin=[]  SaturationOutMax=[]  PParamMin=[]  PParamMax=[]  IParamMin=[]  IParamMax=[]  DParamMin=[]  DParamMax=[]  NParamMin=[]  NParamMax=[]  KbParamMin=[]  KbParamMax=[]  KtParamMin=[]  KtParamMax=[]  KbOutMin=[]  KbOutMax=[]  KtOutMin=[]  KtOutMax=[]  IntegratorOutMin=[]  IntegratorOutMax=[]  FilterOutMin=[]  FilterOutMax=[]  SumI1OutMin=[]  SumI1OutMax=[]  SumI2OutMin=[]  SumI2OutMax=[]  SumI3OutMin=[]  SumI3OutMax=[]  SumI4OutMin=[]  SumI4OutMax=[]  SumDOutMin=[]  SumDOutMax=[]  DifferentiatorOutMin=[]  DifferentiatorOutMax=[]  FilterDiffOutCoefMin=[]  FilterDiffOutCoefMax=[]  ReciprocalOutMin=[]  ReciprocalOutMax=[]  SumDenOutMin=[]  SumDenOutMax=[]  SumNumOutMin=[]  SumNumOutMax=[]  DivideOutMin=[]  DivideOutMax=[]  IntegratorContinuousStateAttributes=''  IntegratorStateMustResolveToSignalObject=off  IntegratorRTWStateStorageClass=Auto  FilterContinuousStateAttributes=''  FilterStateMustResolveToSignalObject=off  FilterRTWStateStorageClass=Auto  ParallelPVariant=InternalParameters  IdealPVariant=Disabled  IVariant=InternalParameters  DVariant=InternalParameters  IntegratorVariant=Discrete  SatVariant=Disabled  AWVariant=Passthrough  PCopyVariant=Disabled  TRVariant=Disabled  FdbkBlocksVariant=Forward  IdealPFdbkVariant=Disabled  SatFdbkVariant=Disabled  DerivativeFilterVariant=ForwardEulerFilter  NVariant=InternalParameters  NCopyVariant=Disabled  FilterICVariant=InternalICsFilter  IntegratorICVariant=InternalICs  ExternalResetVariant=Disabled  TRSumVariant=Passthrough  SumFdbkVariant=Disabled  SumVariant=Sum_PID
  Sum : Sum  Inputs=-+
  Sum1 : Sum  Inputs=+-
  Aileron : Outport
  wires:
  Demanded Heading/1 -> Sum/2
  Current Heading/1 -> Sum/1
  Sum/1 -> Roll Controller/1
  Roll Controller/1 -> Sum1/1
  Sum1/1 -> Aileron Controller/1
  Aileron Controller/1 -> Aileron/1
  Current Roll Angle/1 -> Sum1/2

== system Copy_of_UAV/Primary Arduino/Flight Control/Model Flight Control/Guidance/Guidance.HDG_Hold.HDG/Heading Hold ==
  Current Heading : Inport
  Demanded Heading : Inport  Port=2
  Current Roll Angle : Inport  Port=3
  Aileron Controller : simulink/Continuous/PID Controller  Controller=PID  Form=Parallel  TimeDomain=Discrete-time  SampleTime=-1  IntegratorMethod=Forward Euler  FilterMethod=Forward Euler  ControllerParametersSource=internal  P=1  I=1  D=0  UseFilter=on  N=100  TunerSelectOption=Transfer Function Based (PID Tuner App)  InitialConditionSource=internal  InitialConditionForIntegrator=0  InitialConditionForFilter=0  DifferentiatorICPrevScaledInput=0  ExternalReset=none  TrackingMode=off  Kt=1  LimitOutput=off  UpperSaturationLimit=inf  LowerSaturationLimit=-inf  LinearizeAsGain=off  AntiWindupMode=none  Kb=1  POutMin=[]  POutMax=[]  IOutMin=[]  IOutMax=[]  DOutMin=[]  DOutMax=[]  NOutMin=[]  NOutMax=[]  SumOutMin=[]  SumOutMax=[]  SaturationOutMin=[]  SaturationOutMax=[]  PParamMin=[]  PParamMax=[]  IParamMin=[]  IParamMax=[]  DParamMin=[]  DParamMax=[]  NParamMin=[]  NParamMax=[]  KbParamMin=[]  KbParamMax=[]  KtParamMin=[]  KtParamMax=[]  KbOutMin=[]  KbOutMax=[]  KtOutMin=[]  KtOutMax=[]  IntegratorOutMin=[]  IntegratorOutMax=[]  FilterOutMin=[]  FilterOutMax=[]  SumI1OutMin=[]  SumI1OutMax=[]  SumI2OutMin=[]  SumI2OutMax=[]  SumI3OutMin=[]  SumI3OutMax=[]  SumI4OutMin=[]  SumI4OutMax=[]  SumDOutMin=[]  SumDOutMax=[]  DifferentiatorOutMin=[]  DifferentiatorOutMax=[]  FilterDiffOutCoefMin=[]  FilterDiffOutCoefMax=[]  ReciprocalOutMin=[]  ReciprocalOutMax=[]  SumDenOutMin=[]  SumDenOutMax=[]  SumNumOutMin=[]  SumNumOutMax=[]  DivideOutMin=[]  DivideOutMax=[]  IntegratorContinuousStateAttributes=''  IntegratorStateMustResolveToSignalObject=off  IntegratorRTWStateStorageClass=Auto  FilterContinuousStateAttributes=''  FilterStateMustResolveToSignalObject=off  FilterRTWStateStorageClass=Auto  ParallelPVariant=InternalParameters  IdealPVariant=Disabled  IVariant=InternalParameters  DVariant=InternalParameters  IntegratorVariant=Discrete  SatVariant=Disabled  AWVariant=Passthrough  PCopyVariant=Disabled  TRVariant=Disabled  FdbkBlocksVariant=Forward  IdealPFdbkVariant=Disabled  SatFdbkVariant=Disabled  DerivativeFilterVariant=ForwardEulerFilter  NVariant=InternalParameters  NCopyVariant=Disabled  FilterICVariant=InternalICsFilter  IntegratorICVariant=InternalICs  ExternalResetVariant=Disabled  TRSumVariant=Passthrough  SumFdbkVariant=Disabled  SumVariant=Sum_PID
  Roll Controller : simulink/Continuous/PID Controller  Controller=PID  Form=Parallel  TimeDomain=Discrete-time  SampleTime=-1  IntegratorMethod=Forward Euler  FilterMethod=Forward Euler  ControllerParametersSource=internal  P=1  I=1  D=0  UseFilter=on  N=100  TunerSelectOption=Transfer Function Based (PID Tuner App)  InitialConditionSource=internal  InitialConditionForIntegrator=0  InitialConditionForFilter=0  DifferentiatorICPrevScaledInput=0  ExternalReset=none  TrackingMode=off  Kt=1  LimitOutput=off  UpperSaturationLimit=inf  LowerSaturationLimit=-inf  LinearizeAsGain=off  AntiWindupMode=none  Kb=1  POutMin=[]  POutMax=[]  IOutMin=[]  IOutMax=[]  DOutMin=[]  DOutMax=[]  NOutMin=[]  NOutMax=[]  SumOutMin=[]  SumOutMax=[]  SaturationOutMin=[]  SaturationOutMax=[]  PParamMin=[]  PParamMax=[]  IParamMin=[]  IParamMax=[]  DParamMin=[]  DParamMax=[]  NParamMin=[]  NParamMax=[]  KbParamMin=[]  KbParamMax=[]  KtParamMin=[]  KtParamMax=[]  KbOutMin=[]  KbOutMax=[]  KtOutMin=[]  KtOutMax=[]  IntegratorOutMin=[]  IntegratorOutMax=[]  FilterOutMin=[]  FilterOutMax=[]  SumI1OutMin=[]  SumI1OutMax=[]  SumI2OutMin=[]  SumI2OutMax=[]  SumI3OutMin=[]  SumI3OutMax=[]  SumI4OutMin=[]  SumI4OutMax=[]  SumDOutMin=[]  SumDOutMax=[]  DifferentiatorOutMin=[]  DifferentiatorOutMax=[]  FilterDiffOutCoefMin=[]  FilterDiffOutCoefMax=[]  ReciprocalOutMin=[]  ReciprocalOutMax=[]  SumDenOutMin=[]  SumDenOutMax=[]  SumNumOutMin=[]  SumNumOutMax=[]  DivideOutMin=[]  DivideOutMax=[]  IntegratorContinuousStateAttributes=''  IntegratorStateMustResolveToSignalObject=off  IntegratorRTWStateStorageClass=Auto  FilterContinuousStateAttributes=''  FilterStateMustResolveToSignalObject=off  FilterRTWStateStorageClass=Auto  ParallelPVariant=InternalParameters  IdealPVariant=Disabled  IVariant=InternalParameters  DVariant=InternalParameters  IntegratorVariant=Discrete  SatVariant=Disabled  AWVariant=Passthrough  PCopyVariant=Disabled  TRVariant=Disabled  FdbkBlocksVariant=Forward  IdealPFdbkVariant=Disabled  SatFdbkVariant=Disabled  DerivativeFilterVariant=ForwardEulerFilter  NVariant=InternalParameters  NCopyVariant=Disabled  FilterICVariant=InternalICsFilter  IntegratorICVariant=InternalICs  ExternalResetVariant=Disabled  TRSumVariant=Passthrough  SumFdbkVariant=Disabled  SumVariant=Sum_PID
  Sum : Sum  Inputs=-+
  Sum1 : Sum  Inputs=+-
  Aileron Command : Outport
  wires:
  Demanded Heading/1 -> Sum/2
  Current Heading/1 -> Sum/1
  Sum/1 -> Roll Controller/1
  Roll Controller/1 -> Sum1/1
  Sum1/1 -> Aileron Controller/1
  Aileron Controller/1 -> Aileron Command/1
  Current Roll Angle/1 -> Sum1/2

== system Copy_of_UAV/Primary Arduino/Flight Control/Real Flight Control/Guidance/Guidance.ALT_Hold.ALT/Altitude Hold ==
  ALT : Inport
  Demanded ALT : Inport  Port=2
  theta : Inport  Port=3
  Elevator Controller : simulink/Continuous/PID Controller  Controller=PID  Form=Parallel  TimeDomain=Discrete-time  SampleTime=-1  IntegratorMethod=Forward Euler  FilterMethod=Forward Euler  ControllerParametersSource=internal  P=1  I=1  D=0  UseFilter=on  N=100  TunerSelectOption=Transfer Function Based (PID Tuner App)  InitialConditionSource=internal  InitialConditionForIntegrator=0  InitialConditionForFilter=0  DifferentiatorICPrevScaledInput=0  ExternalReset=none  TrackingMode=off  Kt=1  LimitOutput=off  UpperSaturationLimit=inf  LowerSaturationLimit=-inf  LinearizeAsGain=off  AntiWindupMode=none  Kb=1  POutMin=[]  POutMax=[]  IOutMin=[]  IOutMax=[]  DOutMin=[]  DOutMax=[]  NOutMin=[]  NOutMax=[]  SumOutMin=[]  SumOutMax=[]  SaturationOutMin=[]  SaturationOutMax=[]  PParamMin=[]  PParamMax=[]  IParamMin=[]  IParamMax=[]  DParamMin=[]  DParamMax=[]  NParamMin=[]  NParamMax=[]  KbParamMin=[]  KbParamMax=[]  KtParamMin=[]  KtParamMax=[]  KbOutMin=[]  KbOutMax=[]  KtOutMin=[]  KtOutMax=[]  IntegratorOutMin=[]  IntegratorOutMax=[]  FilterOutMin=[]  FilterOutMax=[]  SumI1OutMin=[]  SumI1OutMax=[]  SumI2OutMin=[]  SumI2OutMax=[]  SumI3OutMin=[]  SumI3OutMax=[]  SumI4OutMin=[]  SumI4OutMax=[]  SumDOutMin=[]  SumDOutMax=[]  DifferentiatorOutMin=[]  DifferentiatorOutMax=[]  FilterDiffOutCoefMin=[]  FilterDiffOutCoefMax=[]  ReciprocalOutMin=[]  ReciprocalOutMax=[]  SumDenOutMin=[]  SumDenOutMax=[]  SumNumOutMin=[]  SumNumOutMax=[]  DivideOutMin=[]  DivideOutMax=[]  IntegratorContinuousStateAttributes=''  IntegratorStateMustResolveToSignalObject=off  IntegratorRTWStateStorageClass=Auto  FilterContinuousStateAttributes=''  FilterStateMustResolveToSignalObject=off  FilterRTWStateStorageClass=Auto  ParallelPVariant=InternalParameters  IdealPVariant=Disabled  IVariant=InternalParameters  DVariant=InternalParameters  IntegratorVariant=Discrete  SatVariant=Disabled  AWVariant=Passthrough  PCopyVariant=Disabled  TRVariant=Disabled  FdbkBlocksVariant=Forward  IdealPFdbkVariant=Disabled  SatFdbkVariant=Disabled  DerivativeFilterVariant=ForwardEulerFilter  NVariant=InternalParameters  NCopyVariant=Disabled  FilterICVariant=InternalICsFilter  IntegratorICVariant=InternalICs  ExternalResetVariant=Disabled  TRSumVariant=Passthrough  SumFdbkVariant=Disabled  SumVariant=Sum_PID
  Pitch Controller : simulink/Continuous/PID Controller  Controller=PID  Form=Parallel  TimeDomain=Discrete-time  SampleTime=-1  IntegratorMethod=Forward Euler  FilterMethod=Forward Euler  ControllerParametersSource=internal  P=1  I=1  D=0  UseFilter=on  N=100  TunerSelectOption=Transfer Function Based (PID Tuner App)  InitialConditionSource=internal  InitialConditionForIntegrator=0  InitialConditionForFilter=0  DifferentiatorICPrevScaledInput=0  ExternalReset=none  TrackingMode=off  Kt=1  LimitOutput=off  UpperSaturationLimit=inf  LowerSaturationLimit=-inf  LinearizeAsGain=off  AntiWindupMode=none  Kb=1  POutMin=[]  POutMax=[]  IOutMin=[]  IOutMax=[]  DOutMin=[]  DOutMax=[]  NOutMin=[]  NOutMax=[]  SumOutMin=[]  SumOutMax=[]  SaturationOutMin=[]  SaturationOutMax=[]  PParamMin=[]  PParamMax=[]  IParamMin=[]  IParamMax=[]  DParamMin=[]  DParamMax=[]  NParamMin=[]  NParamMax=[]  KbParamMin=[]  KbParamMax=[]  KtParamMin=[]  KtParamMax=[]  KbOutMin=[]  KbOutMax=[]  KtOutMin=[]  KtOutMax=[]  IntegratorOutMin=[]  IntegratorOutMax=[]  FilterOutMin=[]  FilterOutMax=[]  SumI1OutMin=[]  SumI1OutMax=[]  SumI2OutMin=[]  SumI2OutMax=[]  SumI3OutMin=[]  SumI3OutMax=[]  SumI4OutMin=[]  SumI4OutMax=[]  SumDOutMin=[]  SumDOutMax=[]  DifferentiatorOutMin=[]  DifferentiatorOutMax=[]  FilterDiffOutCoefMin=[]  FilterDiffOutCoefMax=[]  ReciprocalOutMin=[]  ReciprocalOutMax=[]  SumDenOutMin=[]  SumDenOutMax=[]  SumNumOutMin=[]  SumNumOutMax=[]  DivideOutMin=[]  DivideOutMax=[]  IntegratorContinuousStateAttributes=''  IntegratorStateMustResolveToSignalObject=off  IntegratorRTWStateStorageClass=Auto  FilterContinuousStateAttributes=''  FilterStateMustResolveToSignalObject=off  FilterRTWStateStorageClass=Auto  ParallelPVariant=InternalParameters  IdealPVariant=Disabled  IVariant=InternalParameters  DVariant=InternalParameters  IntegratorVariant=Discrete  SatVariant=Disabled  AWVariant=Passthrough  PCopyVariant=Disabled  TRVariant=Disabled  FdbkBlocksVariant=Forward  IdealPFdbkVariant=Disabled  SatFdbkVariant=Disabled  DerivativeFilterVariant=ForwardEulerFilter  NVariant=InternalParameters  NCopyVariant=Disabled  FilterICVariant=InternalICsFilter  IntegratorICVariant=InternalICs  ExternalResetVariant=Disabled  TRSumVariant=Passthrough  SumFdbkVariant=Disabled  SumVariant=Sum_PID
  Sum : Sum  Inputs=+-
  Sum1 : Sum  Inputs=+-
  Elevator : Outport
  wires:
  Pitch Controller/1 -> Sum1/1
  theta/1 -> Sum1/2
  Demanded ALT/1 -> Sum/2
  Sum/1 -> Pitch Controller/1
  Elevator Controller/1 -> Elevator/1  "Elevator"
  ALT/1 -> Sum/1
  Sum1/1 -> Elevator Controller/1

== system Copy_of_UAV/Primary Arduino/Flight Control/Real Flight Control/Guidance/Guidance.HDG_ALT_Hold.HDG_ALT/Altitude Hold ==
  ALT : Inport
  ALT Demand : Inport  Port=2
  theta : Inport  Port=3
  Altitude Hold : Subsystem
  Elevator : Outport
  wires:
  theta/1 -> Altitude Hold/3(theta)
  ALT Demand/1 -> Altitude Hold/2(In2)
  ALT/1 -> Altitude Hold/1(In1)
  Altitude Hold/1(Elevator) -> Elevator/1
